simulink model "Uncoupled_Aircraft_State_Space"  (R2024b)
settings: Solver=VariableStepAuto  StartTime=0.0  StopTime=600  RelTol=1e-3
values from neighbouring files (symbols this model uses):
  A_lat = [ ... (first row only)    [Rigid_Aircraft_Simulink_Initializer.m]    (also in initialize_plane.m)
  A_long = [ ... (first row only)    [Rigid_Aircraft_Simulink_Initializer.m]    (also in initialize_plane.m)
  B_lat = [ B_ail , B_rud]    [Rigid_Aircraft_Simulink_Initializer.m]    (also in initialize_plane.m)
  B_long = [  B_elv , B_thr ]    [Rigid_Aircraft_Simulink_Initializer.m]    (also in initialize_plane.m)
  const_wind_vector = [6;0;0]    [Rigid_Aircraft_Simulink_Initializer.m]    (also in initialize_plane.m)
  energy_factor_lookup = readmatrix('Energy_Factor_Lookup.csv')    [Rigid_Aircraft_Simulink_Initializer.m]    (also in initialize_plane.m)
  init_alt = 20    [Rigid_Aircraft_Simulink_Initializer.m]    (also in initialize_plane.m = 60)
  init_lat = 52    [Rigid_Aircraft_Simulink_Initializer.m]    (also in initialize_plane.m = 51)
  init_long = 0    [Rigid_Aircraft_Simulink_Initializer.m]    (also in initialize_plane.m)
  L1 = 100    [Rigid_Aircraft_Simulink_Initializer.m]    (also in initialize_plane.m)
  L_day = 25    [Rigid_Aircraft_Simulink_Initializer.m]    (also in initialize_plane.m = 27)
  L_hr = 8    [Rigid_Aircraft_Simulink_Initializer.m]    (also in initialize_plane.m)
  L_month = 8    [Rigid_Aircraft_Simulink_Initializer.m]    (also in initialize_plane.m)
  L_year = 2025    [Rigid_Aircraft_Simulink_Initializer.m]    (also in initialize_plane.m)
  lap_tog = 0    [Rigid_Aircraft_Simulink_Initializer.m]    (also in initialize_plane.m)
  laps = 1    [Rigid_Aircraft_Simulink_Initializer.m]    (also in initialize_plane.m = 10)
  max_cap = 3600*236.80    (= 852480)    [Rigid_Aircraft_Simulink_Initializer.m]    (also in initialize_plane.m)
  max_power_income = 1100*0.18*0.46208    (= 91.49184)    [Rigid_Aircraft_Simulink_Initializer.m]    (also in initialize_plane.m)
  MG = readmatrix('METEO_data.csv')    [Rigid_Aircraft_Simulink_Initializer.m]    (also in initialize_plane.m)
  MGs1 = nan(nlat, nlon, ntime)    [Rigid_Aircraft_Simulink_Initializer.m]    (also in initialize_plane.m)
  MGs2 = nan(nlat, nlon, ntime)    [Rigid_Aircraft_Simulink_Initializer.m]    (also in initialize_plane.m)
  MGs3 = nan(nlat, nlon, ntime)    [Rigid_Aircraft_Simulink_Initializer.m]    (also in initialize_plane.m)
  MGs4 = nan(nlat, nlon, ntime)    [Rigid_Aircraft_Simulink_Initializer.m]    (also in initialize_plane.m)
  MGs5 = nan(nlat, nlon, ntime)    [Rigid_Aircraft_Simulink_Initializer.m]    (also in initialize_plane.m)
  MGs6 = nan(nlat, nlon, ntime)    [Rigid_Aircraft_Simulink_Initializer.m]    (also in initialize_plane.m)
  motor_power = 300    [Rigid_Aircraft_Simulink_Initializer.m]    (also in initialize_plane.m)
  u_trim = xu_trim(5:6)    [Rigid_Aircraft_Simulink_Initializer.m]    (also in initialize_plane.m)
  wind_tog = 1    [Rigid_Aircraft_Simulink_Initializer.m]    (also in initialize_plane.m)
  wind_type = 1    [Rigid_Aircraft_Simulink_Initializer.m]    (also in initialize_plane.m)
  wp_rad = 50    [Rigid_Aircraft_Simulink_Initializer.m]    (also in initialize_plane.m)
  wpts = wpts + zeros(6,1)    [A_star_IP.m]    (also in Rigid_Aircraft_Simulink_Initializer.m = wpts(:,2:end))
  X_eq = [U_inf; 0; 0; Theta_eq]    [Rigid_Aircraft_Simulink_Initializer.m]    (also in initialize_plane.m)
undefined symbols (not defined in the file or in its folder): Alt, aspd_min, gravity, H_INIT, K_D, K_H, K_T, K_V, mass, PTCH2SRV_D, PTCH2SRV_RLL, PTCH2SRV_RMAX_DN, PTCH2SRV_RMAX_UP, PTCH2SRV_TCONST, PTCH_K_I, PTCH_K_P, RLL2SRV_D, RLL2SRV_MAX, RLL2SRV_TCONST, RLL_K_I, RLL_K_P, V_INIT, YAW2SRV_DAMP, YAW2SRV_INT, YAW2SRV_RLL, YAW2SRV_SLIP
libraries: simulink_extras x19, eeGeneralControl x3, dspsrcs4 x3, dspswit3 x2, slpidlib x1, dspstat3 x1, simulink x1
settings Model: Creator=sh2323  LastModifiedBy=sh2323

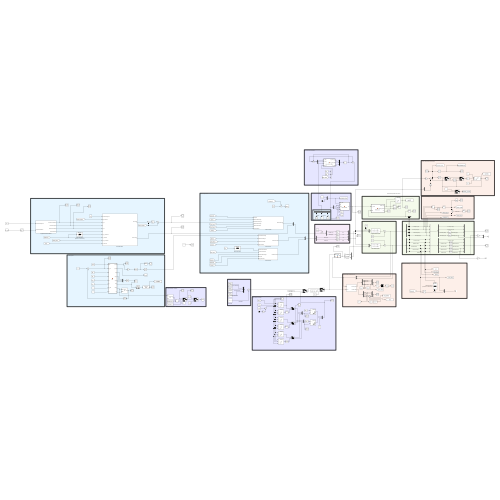
[thumbnail: Simulink's stored preview of the top-level diagram]
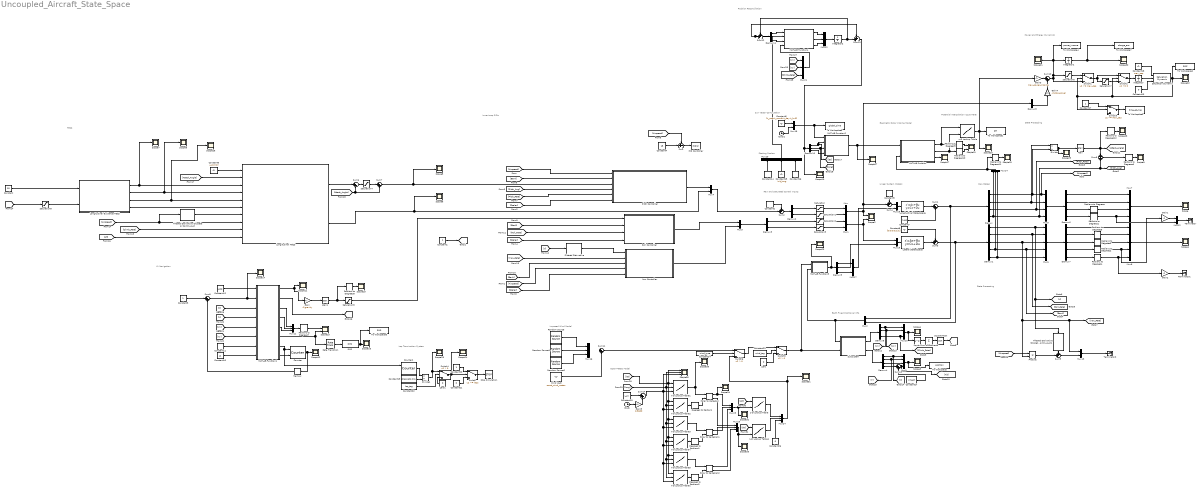
== system Uncoupled_Aircraft_State_Space ==
  note: Potential Interpolation Issue Here!
  note: Open-Meteo Model
  note: Imposed Wind Model
  note: Position Reconciliation
  note: Starting Positon
  note: Power and Energy Dynamics
  note: Lap Termination System
  note: Sun Vector Computation
  note: Geometric Solar Income Model
  note: L1 Navigation
  note: State Processing
  note: State Processing
  note: TECS
  note: Earth Fixed Positional Info
  note: Inner Loop PIDs
  note: Linear System Models
  note: Raw States
  note: Raw and Saturated Control Inputs
  1-D Lookup Table : Lookup_n-D  NumberOfTableDimensions=1  BreakpointsForDimension1=[10;80;120]  TableSource=Input port  Table=Alt  InterpMethod=Cubic spline  ExtrapMethod=Clip  InternalRulePriority=Speed  RndMeth=Simplest
      settings: InputPortMap=u0,p221
  1-D Lookup Table1 : Lookup_n-D  NumberOfTableDimensions=1  BreakpointsForDimension1=[10;80;120]  TableSource=Input port  Table=Alt  InterpMethod=Cubic spline  ExtrapMethod=Clip  InternalRulePriority=Speed  RndMeth=Simplest
      settings: InputPortMap=u0,p221
  Atan : Trigonometry  Operator=atan
  Atan1 : Trigonometry  Operator=atan
  Clock : Clock
  Clock1 : Clock
  Constant : Constant  Value=15
  Constant{1,3,17,20} (4 alike) : Constant
  Constant10 : Constant  Value=L1
  Constant11 : Constant  Value=wp_rad
  Constant12 : Constant  Value=wpts  VectorParams1D=off
  Constant13 : Constant  Value=0
  Constant14 : Constant  Value=init_lat
  Constant15 : Constant  Value=init_long
  Constant16 : Constant  Value=init_alt
  Constant18 : Constant  Value=max_cap
  Constant19 : Constant  Value=size(wpts,2)-1
  Constant2 : Constant  Value=u_trim
  Constant21 : Constant  Value=0
  Constant22 : Constant  Value=lap_tog
  Constant23 : Constant  Value=wind_tog
  Constant24 : Constant  Value=wind_type
  Constant25 : Constant  Value=L_hr
  Constant26 : Constant  Value=0
  Constant27 : Constant  Value=init_alt
  Constant4 : Constant  Value=15
  Constant5 : Constant  Value=[L_year;L_month;L_day;L_hr;0]
  Constant6 : Constant  Value=u_trim(2)
  Constant7 : Constant  Value=X_eq
  Constant8 : Constant  Value=[0;0;0;0;pi/2]
  Constant9 : Constant  Value=u_trim
  Counter : dspswit3/Counter  Direction=Up  CountEvent=Rising edge  CounterSize=User defined  MaxCount=255  InitialCount=0  Output=Count  HitValue=32  ResetInput=on  SamplesPerFrame=1  Ts=1  CntDtype=double  HitDtype=Logical
  Counter1 : dspswit3/Counter  Direction=Up  CountEvent=Rising edge  CounterSize=User defined  MaxCount=255  InitialCount=0  Output=Count  HitValue=32  ResetInput=on  SamplesPerFrame=1  Ts=1  CntDtype=double  HitDtype=Logical
  Degrees to Radians : simulink_extras/Transformations/Degrees to Radians
  Degrees to Radians1 : simulink_extras/Transformations/Degrees to Radians
  Degrees to Radians2 : simulink_extras/Transformations/Degrees to Radians
  Demux{,4..6} (4 alike) : Demux
  Demux1 : Demux  Outputs=5
  Demux10 : Demux  Outputs=3
  Demux11 : Demux  Outputs=3
  Demux2 : Demux  Outputs=2
  Demux3 : Demux  Outputs=2
  Demux7 : Demux  Outputs=5
  Demux8 : Demux  Outputs=2
  Demux9 : Demux  Outputs=3
  Divide : Product  Inputs=*/
  Divide1 : Product  Inputs=*/
  "Filtered Derivative " : eeGeneralControl/Filtered Derivative (Discrete or Continuous)  K=1  T=0.1  B=inf  A=-inf  minRatio=10  init_option=Inherited from block input  x0=0  Ts=-1
      settings: LibrarySourceBlock=|
      | ee_sl_lib/General Control/Filtered Derivative
      | (Discrete or Continuous)
  Filtered Derivative (Discrete or Continuous) : eeGeneralControl/Filtered Derivative (Discrete or Continuous)  K=1  T=0.1  B=inf  A=-inf  minRatio=10  init_option=Inherited from block input  x0=0  Ts=-1
      settings: LibrarySourceBlock=|
      | ee_sl_lib/General Control/Filtered Derivative
      | (Discrete or Continuous)
  Filtered Derivative (Discrete or Continuous)1 : eeGeneralControl/Filtered Derivative (Discrete or Continuous)  K=1  T=0.1  B=inf  A=-inf  minRatio=10  init_option=Inherited from block input  x0=0  Ts=-1
      settings: LibrarySourceBlock=|
      | ee_sl_lib/General Control/Filtered Derivative
      | (Discrete or Continuous)
  Gain : Gain  Gain=-1/gravity
  Gain1 : Gain  Gain=-1
  Gain2 : Gain  Gain=-1
  Gain3 : Gain  Gain=max_power_income
  Gain4 : Gain  Gain=-motor_power
  Gain5 : Gain  Gain=1/3600
  Integrator : Integrator  InitialCondition=max_cap
  Integrator1 : Integrator
  Integrator2 : Integrator
  Lateral State-Space : StateSpace  A=A_lat  B=[B_lat A_lat(:,1)]  C=eye(5)  D=zeros(size([B_lat A_lat(:,1)]))  InitialCondition=0
  Longitudinal Guidance TECS : Subsystem
  Longitudinal State-Space : StateSpace  A=A_long  B=[B_long A_long(:,1:2)]  C=eye(4)  D=zeros(size([B_long A_long(:,1:2)]))  InitialCondition=0
  Longitudinal TECS : Subsystem
  MATLAB Function : MATLAB Function  TreatAsAtomicUnit=on
  MATLAB Function1 : MATLAB Function  TreatAsAtomicUnit=on
  MATLAB Function2 : MATLAB Function  TreatAsAtomicUnit=on
  MATLAB Function3 : MATLAB Function  TreatAsAtomicUnit=on
  MATLAB Function4 : MATLAB Function  TreatAsAtomicUnit=on
  Memory : Memory
  Mux{,1..4,12..13,15,17..19} (11 alike) : Mux  Inputs=2
  Mux{5,7,9..10} (4 alike) : Mux
  Mux{11,14,16,20..25} (9 alike) : Mux  Inputs=3
  Mux6 : Mux  Inputs=5
  Mux8 : Mux  Inputs=5
  PID Controller : slpidlib/PID Controller  Controller=PID  Form=Parallel  TimeDomain=Continuous-time  UseExternalTs=off  SampleTime=-1  IntegratorMethod=Forward Euler  FilterMethod=Forward Euler  ControllerParametersSource=internal  P=1  I=1  UseKiTs=off  D=0  UseExternalDerivativeSource=off  N=100  UseFilter=on  TunerSelectOption=Transfer Function Based (PID Tuner App)  InitialConditionSource=internal  InitialConditionForIntegrator=0  InitialConditionForFilter=0  DifferentiatorICPrevScaledInput=0  ExternalReset=none  TrackingMode=off  Kt=1  LimitOutput=off  SatLimitsSource=internal  UpperSaturationLimit=inf  LowerSaturationLimit=-inf  LinearizeAsGain=on  AntiWindupMode=none  Kb=1  LimitIntegrator=off  UpperIntegratorSaturationLimit=inf  LowerIntegratorSaturationLimit=-inf  POutMin=[]  POutMax=[]  IOutMin=[]  IOutMax=[]  DOutMin=[]  DOutMax=[]  NOutMin=[]  NOutMax=[]  SumOutMin=[]  SumOutMax=[]  SaturationOutMin=[]  SaturationOutMax=[]  PParamMin=[]  PParamMax=[]  IParamMin=[]  IParamMax=[]  DParamMin=[]  DParamMax=[]  NParamMin=[]  NParamMax=[]  KbParamMin=[]  KbParamMax=[]  KtParamMin=[]  KtParamMax=[]  KbOutMin=[]  KbOutMax=[]  KtOutMin=[]  KtOutMax=[]  IntegratorOutMin=[]  IntegratorOutMax=[]  FilterOutMin=[]  FilterOutMax=[]  SumI1OutMin=[]  SumI1OutMax=[]  SumI2OutMin=[]  SumI2OutMax=[]  SumI3OutMin=[]  SumI3OutMax=[]  SumI4OutMin=[]  SumI4OutMax=[]  SumDOutMin=[]  SumDOutMax=[]  DifferentiatorOutMin=[]  DifferentiatorOutMax=[]  FilterDiffOutCoefMin=[]  FilterDiffOutCoefMax=[]  ReciprocalOutMin=[]  ReciprocalOutMax=[]  SumDenOutMin=[]  SumDenOutMax=[]  SumNumOutMin=[]  SumNumOutMax=[]  DivideOutMin=[]  DivideOutMax=[]  UdiffTsProdOutMin=[]  UdiffTsProdOutMax=[]  NTsProdOutMin=[]  NTsProdOutMax=[]  UintegralTsProdOutMin=[]  UintegralTsProdOutMax=[]  UngainTsProdOutMin=[]  UngainTsProdOutMax=[]  ClampingZeroOutDataTypeStr=Inherit: Inherit via back propagation  ClampingZeroOutMin=[]  ClampingZeroOutMax=[]  FilterDenConstantOutDataTypeStr=Inherit: Inherit via back propagation  FilterDenConstantOutMin=[]  FilterDenConstantOutMax=[]  PCopyOutDataTypeStr=Inherit: Inherit via back propagation  PCopyOutMin=[]  PCopyOutMax=[]  NCopyOutDataTypeStr=Inherit: Inherit via back propagation  NCopyOutMin=[]  NCopyOutMax=[]  IntegratorContinuousStateAttributes=''  IntegratorStateMustResolveToSignalObject=off  IntegratorRTWStateStorageClass=Auto  FilterContinuousStateAttributes=''  FilterStateMustResolveToSignalObject=off  FilterRTWStateStorageClass=Auto  ParallelPVariant=InternalParameters  IdealPVariant=Disabled  IVariant=InternalParameters  DVariant=InternalParameters  IntegratorVariant=Continuous  SatVariant=Disabled  AWVariant=Passthrough  PCopyVariant=Disabled  TRVariant=Disabled  FdbkBlocksVariant=Forward  IdealPFdbkVariant=Disabled  SatFdbkVariant=Disabled  DerivativeFilterVariant=ContFilter  NVariant=InternalParameters  NCopyVariant=Disabled  FilterICVariant=InternalICsFilter  IntegratorICVariant=InternalICs  ExternalResetVariant=Disabled  TRSumVariant=Passthrough  SumFdbkVariant=Disabled  SumVariant=Sum_PID  TsampFilterVariant=InternalTs  TsampNgainVariant=Passthrough  TsampIntegralVariant=Disabled_SignalSpec  ExternalSaturationOutDataTypeStr=Inherit: Same as second input  DerivativeSourceVariant=ErrorSignal  PreIntVariant=InternalPreInt
  Pitch Controller : Subsystem
  Polar to Cartesian : simulink_extras/Transformations/Polar to Cartesian
  Polar to Cartesian1 : simulink_extras/Transformations/Polar to Cartesian
  Polar to Cartesian2 : simulink_extras/Transformations/Polar to Cartesian
  Product : Product
  RMS : dspstat3/RMS  run=on  directionMode=Each column  dimension=1  InputProcessing=Columns as channels (frame based)  reset_popup=None
  Radians to Degrees{,1..12} (13 alike) : simulink_extras/Transformations/Radians to Degrees
  Random Source : dspsrcs4/Random Source  SrcType=Gaussian  MinVal=0  MaxVal=1  MeanVal=0  VarVal=0  RepMode=Specify seed  rawSeed=1  IsInherit=off  SampTime=0.25  SampFrame=1  OutComplex=Real  DataType=double  SimulateUsing=Interpreted execution
  Random Source1 : dspsrcs4/Random Source  SrcType=Gaussian  MinVal=0  MaxVal=1  MeanVal=0  VarVal=0.1  RepMode=Specify seed  rawSeed=1  IsInherit=off  SampTime=0.25  SampFrame=1  OutComplex=Real  DataType=double  SimulateUsing=Interpreted execution
  Random Source2 : dspsrcs4/Random Source  SrcType=Gaussian  MinVal=0  MaxVal=1  MeanVal=0  VarVal=0.01  RepMode=Specify seed  rawSeed=1  IsInherit=off  SampTime=0.25  SampFrame=1  OutComplex=Real  DataType=double  SimulateUsing=Interpreted execution
  Rate Transition : RateTransition  OutPortSampleTime=0.05
  Roll Controller : Subsystem
  Saturation : Saturate  UpperLimit=1  LowerLimit=-1
  Saturation Dynamic : simulink/Discontinuities/Saturation Dynamic  OutMin=[]  OutMax=[]  OutDataTypeStr=Inherit: Same as second input  OutDataType=fixdt(1, 16)  OutScaling=2^-10  DoSatur=off
  Saturation1 : Saturate  UpperLimit=1  LowerLimit=0
  Saturation2 : Saturate  UpperLimit=1  LowerLimit=-1
  Saturation3 : Saturate  UpperLimit=1  LowerLimit=-1
  Saturation4 : Saturate  UpperLimit=deg2rad(10)  LowerLimit=deg2rad(-10)
  Saturation5 : Saturate  UpperLimit=deg2rad(30)  LowerLimit=-deg2rad(30)
  Saturation6 : Saturate  UpperLimit=0  LowerLimit=-inf
  Saturation7 : Saturate  UpperLimit=inf  LowerLimit=0
  Saturation8 : Saturate  UpperLimit=120  LowerLimit=0
  Scope{,1,3..9,11..12,14..35} (33 alike) : Scope
  Scope10 : Scope  NumInputPorts=2
  Scope13 : Scope  NumInputPorts=2
  Scope2 : Scope  NumInputPorts=2
  Scope36 : Scope  NumInputPorts=3
  Square : Math  Operator=square
  Square Root : Sqrt
  Stop Simulation : Stop
  Subsystem : Subsystem
  Sum : Sum  Inputs=-+|
  Sum of Elements : Sum  Inputs=+
  Sum{1,7..8,10..11,14..15} (7 alike) : Sum  Inputs=|++
  Sum{2..3,9,12..13} (5 alike) : Sum  Inputs=++|
  Sum4 : Sum  Inputs=-+|
  Sum5 : Sum  Inputs=+|+
  Sum6 : Sum  Inputs=|+-
  Switch : Switch  Threshold=laps  SaturateOnIntegerOverflow=off  InputSameDT=off
  Switch1 : Switch  Threshold=max_cap  SaturateOnIntegerOverflow=off  InputSameDT=off
  Switch2 : Switch  SaturateOnIntegerOverflow=off  InputSameDT=off
  Switch3 : Switch  Threshold=max_cap  SaturateOnIntegerOverflow=off  InputSameDT=off
  Switch4 : Switch  Criteria=u2 > Threshold  SaturateOnIntegerOverflow=off  InputSameDT=off
  Switch5 : Switch  Criteria=u2 > Threshold  SaturateOnIntegerOverflow=off  InputSameDT=off
  Switch6 : Switch  Criteria=u2 > Threshold  SaturateOnIntegerOverflow=off  InputSameDT=off
  Terminator : Terminator
  Terminator1 : Terminator
  Terminator2 : Terminator
  To Workspace : ToWorkspace  VariableName=position  SaveFormat=Timeseries  SampleTime=-1
  To Workspace1 : ToWorkspace  VariableName=SFI  SaveFormat=Timeseries  SampleTime=-1
  To Workspace2 : ToWorkspace  VariableName=SOC  SaveFormat=Timeseries  SampleTime=-1
  To Workspace3 : ToWorkspace  VariableName=time_at_max  SaveFormat=Timeseries  SampleTime=-1
  To Workspace4 : ToWorkspace  VariableName=power_income  SaveFormat=Timeseries  SampleTime=-1
  To Workspace5 : ToWorkspace  VariableName=global_time  SaveFormat=Timeseries  SampleTime=-1
  To Workspace6 : ToWorkspace  VariableName=RMS  SaveFormat=Timeseries  SampleTime=-1
  To Workspace7 : ToWorkspace  VariableName=charge_acc  SaveFormat=Timeseries  SampleTime=-1
  Wind Vect : Constant  Value=const_wind_vector
  Yaw Controller : Subsystem
  Zero : Constant  Value=0  OutDataTypeStr=Inherit: Inherit via back propagation
  Zero1 : Constant  Value=0  OutDataTypeStr=Inherit: Inherit via back propagation
  n-D Lookup Table : Lookup_n-D  BreakpointsForDimension1=unique(energy_factor_lookup(:,1))  BreakpointsForDimension2=unique(energy_factor_lookup(:,2))  BreakpointsForDimension3=[5, 7]  Table=Z'  ExtrapMethod=Clip  InternalRulePriority=Speed  RndMeth=Simplest
      settings: InputPortMap=u0,u1
  n-D Lookup Table1 : Lookup_n-D  NumberOfTableDimensions=3  BreakpointsForDimension1=unique(MG(:,1))  BreakpointsForDimension2=unique(MG(:,2))  BreakpointsForDimension3=unique(MG(:,3))  Table=MGs1  InterpMethod=Cubic spline  ExtrapMethod=Clip  InternalRulePriority=Speed  RndMeth=Simplest
      settings: InputPortMap=u0,u1,u2
  n-D Lookup Table2 : Lookup_n-D  NumberOfTableDimensions=3  BreakpointsForDimension1=unique(MG(:,1))  BreakpointsForDimension2=unique(MG(:,2))  BreakpointsForDimension3=unique(MG(:,3))  Table=MGs2  InterpMethod=Cubic spline  ExtrapMethod=Clip  InternalRulePriority=Speed  RndMeth=Simplest
      settings: InputPortMap=u0,u1,u2
  n-D Lookup Table3 : Lookup_n-D  NumberOfTableDimensions=3  BreakpointsForDimension1=unique(MG(:,1))  BreakpointsForDimension2=unique(MG(:,2))  BreakpointsForDimension3=unique(MG(:,3))  Table=MGs3  InterpMethod=Cubic spline  ExtrapMethod=Clip  InternalRulePriority=Speed  RndMeth=Simplest
      settings: InputPortMap=u0,u1,u2
  n-D Lookup Table4 : Lookup_n-D  NumberOfTableDimensions=3  BreakpointsForDimension1=unique(MG(:,1))  BreakpointsForDimension2=unique(MG(:,2))  BreakpointsForDimension3=unique(MG(:,3))  Table=MGs4  InterpMethod=Cubic spline  ExtrapMethod=Clip  InternalRulePriority=Speed  RndMeth=Simplest
      settings: InputPortMap=u0,u1,u2
  n-D Lookup Table5 : Lookup_n-D  NumberOfTableDimensions=3  BreakpointsForDimension1=unique(MG(:,1))  BreakpointsForDimension2=unique(MG(:,2))  BreakpointsForDimension3=unique(MG(:,3))  Table=MGs5  InterpMethod=Cubic spline  ExtrapMethod=Clip  InternalRulePriority=Speed  RndMeth=Simplest
      settings: InputPortMap=u0,u1,u2
  n-D Lookup Table6 : Lookup_n-D  NumberOfTableDimensions=3  BreakpointsForDimension1=unique(MG(:,1))  BreakpointsForDimension2=unique(MG(:,2))  BreakpointsForDimension3=unique(MG(:,3))  Table=MGs6  InterpMethod=Cubic spline  ExtrapMethod=Clip  InternalRulePriority=Speed  RndMeth=Simplest
      settings: InputPortMap=u0,u1,u2
  wires:
  Demux7/5 -> Radians to Degrees4/1  "Heading (rad)"
  Demux1/5 -> Mux6/5, Mux14/3  "Heading (rad)"
  Mux6/1 -> Demux7/1
  Demux6/1 -> Mux7/1  "X-velocity U (m/s)"
  Demux/3 -> Mux5/3, [Pitch_Rate]  "Pitch Rate (rad/s)"
  Demux7/2 -> Radians to Degrees5/1  "Roll Rate (rad/s)"
  Radians to Degrees2/1 -> Gain1/1, Mux8/4  "Bank Angle (deg)"
  Mux5/1 -> Demux6/1
  Demux/4 -> Sum5/2, [Pitch_Ang], Mux5/4, Mux14/1  "Pitch Angle (rad)"
  Demux6/4 -> Radians to Degrees1/1  "Pitch Angle (rad)"
  Demux7/3 -> Radians to Degrees3/1  "Yaw Rate (rad/s)"
  Demux/2 -> Divide/1, Mux5/2  "Z-velocity  W (m/s)"
  Demux7/1 -> Mux8/1  "Y-velocity V (m/s)"
  Radians to Degrees/1 -> Mux7/3  "Pitch Rate (deg/s)"
  Demux1/2 -> [Roll_Rate], Mux6/2  "Roll Rate (rad/s)"
  Demux/1 -> Divide/2, [Airspeed], Mux5/1  "X-velocity U (m/s)"
  Radians to Degrees4/1 -> Gain2/1, Mux8/5  "Heading (deg)"
  Demux7/4 -> Radians to Degrees2/1  "Bank Angle (rad)"
  Demux1/1 -> [V], Filtered Derivative (Discrete or Continuous)1/1, Mux6/1  "Y-velocity V (m/s)"
  Radians to Degrees5/1 -> Mux8/2  "Roll Rate (deg/s)"
  Demux1/3 -> Product/2, Mux13/1, [Yaw_Rate], Mux6/3  "Yaw Rate (rad/s)"
  Demux6/3 -> Radians to Degrees/1  "Pitch Rate (rad/s)"
  Demux6/2 -> Mux7/2  "Z-velocity  W (m/s)"
  Mux8/1 -> Scope1/1
  Mux7/1 -> Scope/1
  Demux1/4 -> [Bank], Mux6/4, Mux14/2  "Bank Angle (rad)"
  Radians to Degrees3/1 -> Mux8/3  "Yaw Rate (deg/s)"
  Radians to Degrees1/1 -> Mux12/2, Mux7/4  "Pitch Angle (deg)"
  Lateral State-Space/1 -> Sum3/2
  Demux3/2 -> Saturation3/1  "Rudder(%)"
  Saturation1/1 -> Mux/2  "Thr"
  Saturation/1 -> Mux/1  "Elv"
  Demux2/1 -> Saturation/1  "Elelvator (%)"
  Demux3/1 -> Saturation2/1  "Aileron (%)"
  Saturation2/1 -> Mux1/1  "Ail"
  Demux2/2 -> Saturation1/1  "Throttle (%)"
  Saturation3/1 -> Mux1/2  "Rud"
  Mux/1 -> Sum4/2, Demux8/1, Scope2/1
  Mux1/1 -> Mux19/1, Scope2/2
  Sum2/1 -> Demux2/1
  Longitudinal State-Space/1 -> Sum1/1
  Mux2/1 -> MATLAB Function3/2(X), Subsystem/1(X)
  Mux4/1 -> Sum2/2
  Mux3/1 -> Demux3/1
  Roll Controller/1(Aileron Demand) -> Mux3/1
  Yaw Controller/1(Rudder Demand) -> Mux3/2
  "Filtered Derivative "/1 -> Yaw Controller/1(Measured Acceleration)
  Sum/1 -> PID Controller/1
  Constant4/1 -> Sum/2
  Pitch Controller/1(Elevator Demand) -> Mux4/1
  Longitudinal Guidance TECS/4(Desired Altitude) -> Longitudinal TECS/6(h)
  Longitudinal Guidance TECS/3(Desired Climb Rate) -> Scope26/1, Longitudinal TECS/5(h_dot)
  [Climb_Rate] -> Longitudinal TECS/9(h_dot_measured)
  Longitudinal Guidance TECS/2(Desired Airspeed) -> Scope8/1, Longitudinal TECS/4(V)
  Longitudinal Guidance TECS/1(Desired Acceleration) -> Scope7/1, Longitudinal TECS/3(V_dot)
  Constant/1 -> Longitudinal Guidance TECS/1(Commanded Airspeed)
  [Alt] -> Longitudinal TECS/10(h_measured)
  [Airspeed] -> Pitch Controller/1(Airspeed)
  [Airspeed] -> Yaw Controller/4(Airspeed)
  Constant1/1 -> [Scaler]
  [Scaler] -> Pitch Controller/6(Airspeed Scaler)
  [Scaler] -> Roll Controller/4(Airspeed Scaler)
  [Scaler] -> Yaw Controller/5(Airspeed Scaler)
  [Airspeed] -> Sum/1
  [Pitch_Ang] -> Pitch Controller/4(Measured Pitch Angle)
  [Pitch_Rate] -> Pitch Controller/5(Measured Pitch Rate)
  [Bank] -> Pitch Controller/2(Measured Bank Angle)
  [Bank] -> Roll Controller/2(Measured Roll Angle)
  [Bank] -> Yaw Controller/3(Measured Bank Angle)
  [Roll_Rate] -> Roll Controller/3(Measured Roll Rate)
  [V] -> "Filtered Derivative "/1
  [Yaw_Rate] -> Yaw Controller/2(Measured Yaw Rate)
  Sum1/1 -> Mux2/1, Demux/1
  Sum3/1 -> Demux1/1, Mux2/2
  Constant7/1 -> Sum1/2
  Constant8/1 -> Sum3/1
  Constant2/1 -> Sum2/1
  Subsystem/2(Position Vec) -> Demux4/1
  Subsystem/1(Velocity Vec.) -> Demux5/1
  Demux5/1 -> Mux10/1, [Vx]  "X-Velocity (m/s)"
  Demux5/2 -> Mux10/2, [Vy]  "Y-Velocity (m/s)"
  Demux5/4 -> [Climb_Rate], Mux10/4  "Climb Rate (m/s)"
  Mux10/1 -> Square/1, Scope4/1
  Demux4/2 -> [Y], Mux9/2  "Y (m)"
  Mux9/1 -> To Workspace/1, Scope3/1
  Square/1 -> Sum of Elements/1
  Sum of Elements/1 -> Square Root/1
  Square Root/1 -> [V_net]
  [Airspeed] -> Longitudinal TECS/8(V_measured), Filtered Derivative (Discrete or Continuous)/1
  Filtered Derivative (Discrete or Continuous)/1 -> Longitudinal TECS/7(V_dot_measured)
  Divide/1 -> Scope29/1, Atan/1
  Atan/1 -> Radians to Degrees12/1, Sum5/1, [Attack_Angle]
  Longitudinal TECS/2(Thrust Control) -> Scope6/1, Mux4/2
  Longitudinal TECS/1(Pitch Angle) -> Sum6/1
  Sum5/1 -> Radians to Degrees6/1  "Climb Grad."
  Radians to Degrees6/1 -> Scope9/1
  Constant6/1 -> Longitudinal TECS/1(estimated drag force)
  Sum7/1 -> Scope5/1, Pitch Controller/3(Demanded Pitch Angle)
  Sum6/1 -> Saturation4/1
  Saturation4/1 -> Sum7/1
  MATLAB Function1/1(a_cmd) -> Gain/1, Scope11/1
  Constant11/1 -> MATLAB Function1/7(wp_rad)
  Demux4/1 -> [X], Mux9/1  "X (m)"
  [Y] -> MATLAB Function1/4(Y)
  [Vx] -> MATLAB Function1/5(Vx)
  [Vy] -> MATLAB Function1/6(Vy)
  Constant12/1 -> MATLAB Function1/1(wpts)
  Gain/1 -> Atan1/1
  MATLAB Function1/3(ang) -> Mux11/1
  Radians to Degrees7/1 -> Scope13/1
  Radians to Degrees8/1 -> Scope15/1
  Atan1/1 -> Saturation5/1, Radians to Degrees8/1
  Demux4/3 -> Mux9/3
  [X] -> MATLAB Function1/3(X)
  Constant10/1 -> MATLAB Function1/8(L1)
  Counter/1 -> Memory/1, Scope12/1
  MATLAB Function1/7(ticker) -> Counter1/1, Counter/1
  Sum8/1 -> Scope14/1, MATLAB Function1/2(wp_id)
  Constant3/1 -> Sum8/1
  Memory/1 -> Sum8/2
  MATLAB Function1/4(eta_1) -> Mux11/2
  MATLAB Function1/5(eta_2) -> Mux11/3
  Mux11/1 -> Radians to Degrees7/1
  MATLAB Function1/6(CTE) -> Rate Transition/1, Scope13/2
  RMS/1 -> To Workspace6/1, Scope16/1
  Rate Transition/1 -> RMS/1
  Mux12/1 -> Terminator/1
  Gain1/1 -> Mux12/1
  Gain2/1 -> Terminator1/1
  [Airspeed] -> Product/1
  Product/1 -> Sum9/2
  Filtered Derivative (Discrete or Continuous)1/1 -> Sum9/1
  Sum9/1 -> Mux13/2
  Mux13/1 -> Terminator2/1
  MATLAB Function1/2(h_cmd) -> [h_cmd]
  MATLAB Function1/8(rst) -> Counter/2
  MATLAB Function2/1(SI) -> Scope27/1, MATLAB Function/1(sun_vector)
  MATLAB Function/1(relative_elv) -> n-D Lookup Table/1, Radians to Degrees9/1
  MATLAB Function/2(relative_azimuth) -> n-D Lookup Table/2, Radians to Degrees10/1
  Radians to Degrees9/1 -> Scope10/1
  Radians to Degrees10/1 -> Scope10/2
  MATLAB Function/3(vec) -> Scope17/1
  Constant5/1 -> Mux15/1
  Clock1/1 -> Mux15/2
  n-D Lookup Table/1 -> Gain3/1, Scope20/1, To Workspace1/1
  Demux8/2 -> Gain4/1
  Gain4/1 -> Sum10/2
  Gain3/1 -> Sum10/1
  Integrator/1 -> Saturation Dynamic/2
  Saturation Dynamic/1 -> To Workspace2/1, Switch1/2, Switch3/2, Switch2/2, Scope22/1
  Constant13/1 -> Saturation Dynamic/3
  Saturation6/1 -> Switch1/1
  Sum10/1 -> Switch1/3, Scope21/1, To Workspace4/1, Integrator1/1, Saturation6/1
  Switch2/1 -> Integrator/1
  Switch1/1 -> Switch2/1, Saturation7/1
  Saturation7/1 -> Switch2/3
  Constant18/1 -> Saturation Dynamic/1
  Constant17/1 -> Switch3/1
  Switch3/1 -> To Workspace3/1
  Random Source/1 -> Mux16/1  "North wind Noise"
  Random Source1/1 -> Mux16/2  "East Wind Noise"
  Random Source2/1 -> Mux16/3  "Down Wind Noise"
  Wind Vect/1 -> Sum11/2  "NED Wind"
  MATLAB Function3/1(Wind) -> Scope23/1, Demux9/1
  Constant9/1 -> Sum4/1
  Mux18/1 -> Longitudinal State-Space/1
  Sum4/1 -> Mux18/1
  Demux9/1 -> Mux17/1  "U-wind"
  Mux19/1 -> Lateral State-Space/1
  Mux15/1 -> MATLAB Function2/1(time_info), To Workspace5/1
  Constant19/1 -> Divide1/2
  Switch/1 -> Stop Simulation/1
  Constant20/1 -> Switch/1
  Constant21/1 -> Switch/3
  Counter1/1 -> Divide1/1
  Switch4/1 -> Switch/2, Scope24/1
  Constant22/1 -> Switch4/2
  Divide1/1 -> Scope25/1, Switch4/1
  Integrator1/1 -> To Workspace7/1, Scope30/1
  Mux14/1 -> Radians to Degrees11/1, MATLAB Function/2(Euler)
  Radians to Degrees11/1 -> Scope18/1
  Radians to Degrees12/1 -> Scope28/1
  Demux9/2 -> Mux19/2  "V-wind"
  Demux9/3 -> Mux17/2  "W-wind"
  [Attack_Angle] -> Sum7/2, Sum6/2
  [Attack_Angle] -> Longitudinal TECS/2(angle of attack)
  Mux17/1 -> Mux18/2
  Constant14/1 -> Mux20/1  "latitude"
  Constant15/1 -> Mux20/2  "longitude"
  Demux10/1 -> [lat], MATLAB Function2/2(lat)
  Demux10/2 -> [long], MATLAB Function2/3(long)
  Demux10/3 -> MATLAB Function2/4(alt)
  Constant16/1 -> Mux20/3  "alt"
  Saturation5/1 -> Roll Controller/1(Demanded Roll Angle)
  Sum13/1 -> Scope19/1, Demux10/1
  Demux11/3 -> MATLAB Function4/3(h)
  Mux22/1 -> Integrator2/1
  MATLAB Function4/2(lon_rate_deg) -> Mux22/2
  MATLAB Function4/1(lat_rate_deg) -> Mux22/1
  [Vx] -> Mux21/1
  MATLAB Function4/3(h_rate) -> Mux22/3
  [Climb_Rate] -> Mux21/3
  [Vy] -> Mux21/2
  Mux21/1 -> MATLAB Function4/4(neu_vel)
  Integrator2/1 -> Sum13/2, Sum12/1
  Demux11/2 -> MATLAB Function4/2(lon_deg)
  Sum12/1 -> Demux11/1
  Mux20/1 -> Sum13/1, Sum12/2
  Demux11/1 -> MATLAB Function4/1(lat_deg)
  Switch5/1 -> MATLAB Function3/1(Earth_Wind), Subsystem/2(wind)
  Constant23/1 -> Switch5/2
  Switch6/1 -> Switch5/1
  Sum11/1 -> Switch6/1
  Constant24/1 -> Switch6/2
  n-D Lookup Table1/1 -> Scope35/1, Polar to Cartesian/1
  Zero/1 -> Switch5/3
  Zero1/1 -> Switch4/3
  [lat] -> Scope36/1, n-D Lookup Table6/1, n-D Lookup Table5/1, n-D Lookup Table4/1, n-D Lookup Table3/1, n-D Lookup Table2/1, n-D Lookup Table1/1
  [long] -> Scope36/2, n-D Lookup Table6/2, n-D Lookup Table5/2, n-D Lookup Table4/2, n-D Lookup Table3/2, n-D Lookup Table2/2, n-D Lookup Table1/2
  Constant25/1 -> Sum14/1
  Gain5/1 -> Sum14/2
  Clock/1 -> Gain5/1
  Sum14/1 -> Scope36/3, n-D Lookup Table6/3, n-D Lookup Table5/3, n-D Lookup Table4/3, n-D Lookup Table3/3, n-D Lookup Table2/3, n-D Lookup Table1/3
  n-D Lookup Table3/1 -> Polar to Cartesian1/1
  n-D Lookup Table5/1 -> Polar to Cartesian2/1
  Polar to Cartesian/1 -> Scope34/1, Mux23/1
  Polar to Cartesian1/1 -> Mux23/2
  Polar to Cartesian2/1 -> Mux23/3
  1-D Lookup Table/1 -> Mux24/1
  1-D Lookup Table1/1 -> Mux24/2
  Constant26/1 -> Mux24/3
  Polar to Cartesian1/2 -> Mux25/2
  Polar to Cartesian/2 -> Mux25/1
  Polar to Cartesian2/2 -> Mux25/3
  Mux25/1 -> 1-D Lookup Table1/2, Scope33/1
  Mux24/1 -> Scope31/1, Switch6/3
  n-D Lookup Table2/1 -> Degrees to Radians/1
  Degrees to Radians/1 -> Polar to Cartesian/2
  n-D Lookup Table4/1 -> Degrees to Radians1/1
  Degrees to Radians1/1 -> Polar to Cartesian1/2
  n-D Lookup Table6/1 -> Degrees to Radians2/1
  Degrees to Radians2/1 -> Polar to Cartesian2/2
  Mux23/1 -> 1-D Lookup Table/2, Scope32/1
  [Alt] -> 1-D Lookup Table/1
  [Alt] -> 1-D Lookup Table1/1
  Constant27/1 -> Sum15/2
  [h_cmd] -> Saturation8/1
  Saturation8/1 -> Longitudinal Guidance TECS/2(Commanded Altitude)
  Sum15/1 -> [Alt], Mux9/4
  Demux4/4 -> Sum15/1  "Alt (m)"

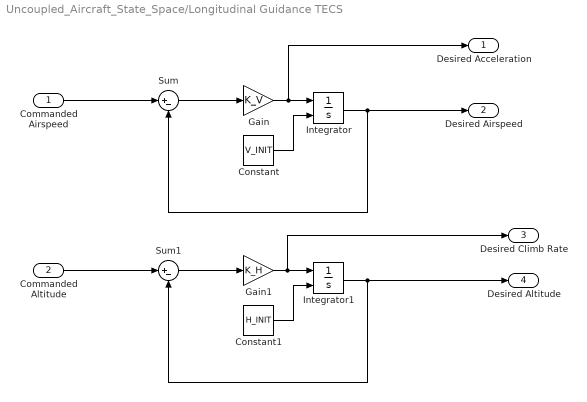
== system Uncoupled_Aircraft_State_Space/Longitudinal Guidance TECS ==
  Commanded Airspeed : Inport
  Commanded Altitude : Inport  Port=2
  Constant : Constant  Value=V_INIT
  Constant1 : Constant  Value=H_INIT
  Gain : Gain  Gain=K_V
  Gain1 : Gain  Gain=K_H
  Integrator : Integrator  InitialConditionSource=external
  Integrator1 : Integrator  InitialConditionSource=external
  Sum : Sum  Inputs=|+-
  Sum1 : Sum  Inputs=|+-
  Desired Acceleration : Outport
  Desired Airspeed : Outport  Port=2
  Desired Climb Rate : Outport  Port=3
  Desired Altitude : Outport  Port=4
  wires:
  Sum/1 -> Gain/1
  Gain/1 -> Desired Acceleration/1, Integrator/1
  Commanded Altitude/1 -> Sum1/1
  Constant/1 -> Integrator/2
  Integrator1/1 -> Desired Altitude/1, Sum1/2
  Gain1/1 -> Desired Climb Rate/1, Integrator1/1
  Commanded Airspeed/1 -> Sum/1
  Integrator/1 -> Desired Airspeed/1, Sum/2
  Constant1/1 -> Integrator1/2
  Sum1/1 -> Gain1/1

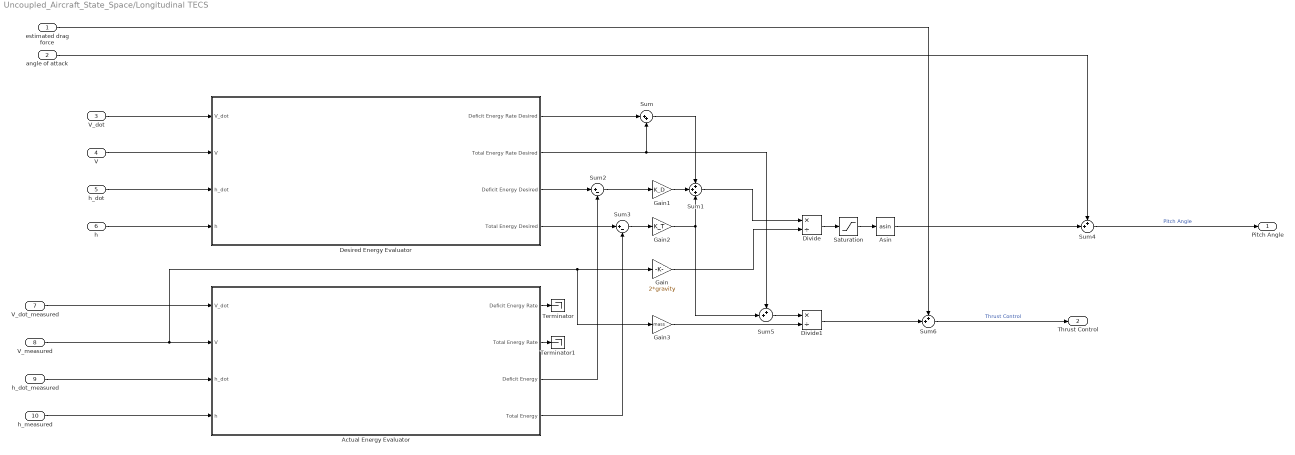
== system Uncoupled_Aircraft_State_Space/Longitudinal TECS ==
  estimated drag force : Inport
  angle of attack : Inport  Port=2
  V_dot : Inport  Port=3
  V : Inport  Port=4
  h_dot : Inport  Port=5
  h : Inport  Port=6
  V_dot_measured : Inport  Port=7
  V_measured : Inport  Port=8
  h_dot_measured : Inport  Port=9
  h_measured : Inport  Port=10
  Actual Energy Evaluator : Subsystem
  Asin : Trigonometry  Operator=asin
  Desired Energy Evaluator : Subsystem
  Divide : Product  Inputs=*/
  Divide1 : Product  Inputs=*/
  Gain : Gain  Gain=2*gravity
  Gain1 : Gain  Gain=K_D
  Gain2 : Gain  Gain=K_T
  Gain3 : Gain  Gain=mass
  Saturation : Saturate  UpperLimit=1  LowerLimit=-1
  Sum : Sum  Inputs=|++
  Sum1 : Sum  Inputs=+++
  Sum2 : Sum  Inputs=|+-
  Sum3 : Sum  Inputs=|+-
  Sum4 : Sum  Inputs=++|
  Sum5 : Sum  Inputs=++|
  Sum6 : Sum  Inputs=++|
  Terminator : Terminator
  Terminator1 : Terminator
  Pitch Angle : Outport
  Thrust Control : Outport  Port=2
  wires:
  Desired Energy Evaluator/2(Total Energy Rate Desired) -> Sum5/1, Sum/2
  Gain2/1 -> Sum5/2, Sum1/3
  angle of attack/1 -> Sum4/1
  Actual Energy Evaluator/3(Deficit Energy) -> Sum2/2
  V/1 -> Desired Energy Evaluator/2(V)
  Desired Energy Evaluator/3(Deficit Energy Desired) -> Sum2/1
  Sum3/1 -> Gain2/1
  V_measured/1 -> Gain3/1, Gain/1, Actual Energy Evaluator/2(V)
  Actual Energy Evaluator/4(Total Energy) -> Sum3/2
  h_dot_measured/1 -> Actual Energy Evaluator/3(h_dot)
  Sum/1 -> Sum1/1
  Gain/1 -> Divide/2
  Desired Energy Evaluator/1(Deficit Energy Rate Desired) -> Sum/1
  Gain3/1 -> Divide1/2
  Actual Energy Evaluator/1(Deficit Energy Rate) -> Terminator/1
  Divide1/1 -> Sum6/2
  Actual Energy Evaluator/2(Total Energy Rate) -> Terminator1/1
  h/1 -> Desired Energy Evaluator/4(h)
  Desired Energy Evaluator/4(Total Energy Desired) -> Sum3/1
  Sum5/1 -> Divide1/1
  Sum2/1 -> Gain1/1
  Saturation/1 -> Asin/1
  Gain1/1 -> Sum1/2
  Sum1/1 -> Divide/1
  V_dot_measured/1 -> Actual Energy Evaluator/1(V_dot)
  h_dot/1 -> Desired Energy Evaluator/3(h_dot)
  estimated drag force/1 -> Sum6/1
  V_dot/1 -> Desired Energy Evaluator/1(V_dot)
  Sum6/1 -> Thrust Control/1  "Thrust Control"
  h_measured/1 -> Actual Energy Evaluator/4(h)
  Sum4/1 -> Pitch Angle/1  "Pitch Angle"
  Divide/1 -> Saturation/1
  Asin/1 -> Sum4/2

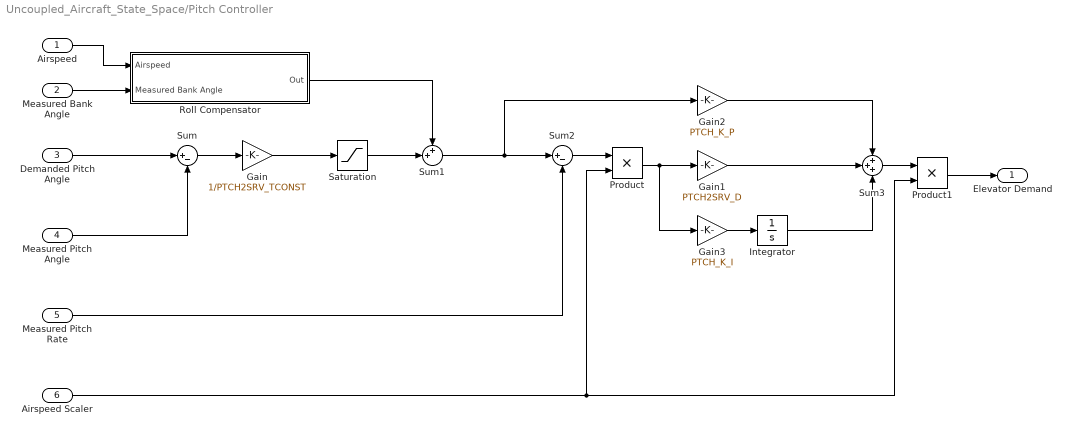
== system Uncoupled_Aircraft_State_Space/Pitch Controller ==
  Airspeed : Inport
  Measured Bank Angle : Inport  Port=2
  Demanded Pitch Angle : Inport  Port=3
  Measured Pitch Angle : Inport  Port=4
  Measured Pitch Rate : Inport  Port=5
  Airspeed Scaler : Inport  Port=6
  Gain : Gain  Gain=1/PTCH2SRV_TCONST
  Gain1 : Gain  Gain=PTCH2SRV_D
  Gain2 : Gain  Gain=PTCH_K_P
  Gain3 : Gain  Gain=PTCH_K_I
  Integrator : Integrator
  Product : Product
  Product1 : Product
  Roll Compensator : Subsystem
  Saturation : Saturate  UpperLimit=PTCH2SRV_RMAX_UP  LowerLimit=PTCH2SRV_RMAX_DN
  Sum : Sum  Inputs=|+-
  Sum1 : Sum  Inputs=++|
  Sum2 : Sum  Inputs=|+-
  Sum3 : Sum  Inputs=+++
  Elevator Demand : Outport
  wires:
  Airspeed/1 -> Roll Compensator/1(Airspeed)
  Gain3/1 -> Integrator/1
  Gain1/1 -> Sum3/2
  Product1/1 -> Elevator Demand/1
  Measured Bank Angle/1 -> Roll Compensator/2(Measured Bank Angle)
  Sum3/1 -> Product1/1
  Measured Pitch Angle/1 -> Sum/2
  Saturation/1 -> Sum1/2
  Sum1/1 -> Gain2/1, Sum2/1
  Product/1 -> Gain3/1, Gain1/1
  Integrator/1 -> Sum3/3
  Demanded Pitch Angle/1 -> Sum/1
  Airspeed Scaler/1 -> Product1/2, Product/2
  Gain/1 -> Saturation/1
  Sum/1 -> Gain/1
  Sum2/1 -> Product/1
  Gain2/1 -> Sum3/1
  Roll Compensator/1(Out) -> Sum1/1
  Measured Pitch Rate/1 -> Sum2/2

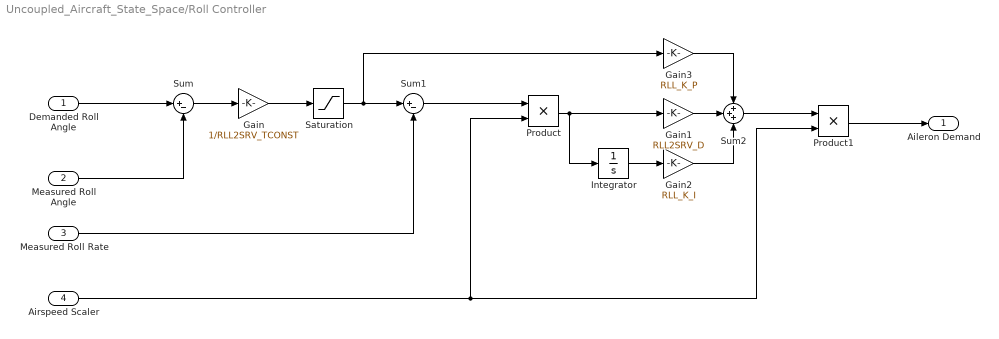
== system Uncoupled_Aircraft_State_Space/Roll Controller ==
  Demanded Roll Angle : Inport
  Measured Roll Angle : Inport  Port=2
  Measured Roll Rate : Inport  Port=3
  Airspeed Scaler : Inport  Port=4
  Gain : Gain  Gain=1/RLL2SRV_TCONST
  Gain1 : Gain  Gain=RLL2SRV_D
  Gain2 : Gain  Gain=RLL_K_I
  Gain3 : Gain  Gain=RLL_K_P
  Integrator : Integrator
  Product : Product
  Product1 : Product
  Saturation : Saturate  UpperLimit=RLL2SRV_MAX  LowerLimit=-RLL2SRV_MAX
  Sum : Sum  Inputs=|+-
  Sum1 : Sum  Inputs=|+-
  Sum2 : Sum  Inputs=+++
  Aileron Demand : Outport
  wires:
  Product/1 -> Integrator/1, Gain1/1
  Sum/1 -> Gain/1
  Saturation/1 -> Sum1/1, Gain3/1
  Gain1/1 -> Sum2/2
  Integrator/1 -> Gain2/1
  Sum2/1 -> Product1/1
  Sum1/1 -> Product/1
  Gain/1 -> Saturation/1
  Gain3/1 -> Sum2/1
  Airspeed Scaler/1 -> Product1/2, Product/2
  Gain2/1 -> Sum2/3
  Demanded Roll Angle/1 -> Sum/1
  Measured Roll Angle/1 -> Sum/2
  Product1/1 -> Aileron Demand/1
  Measured Roll Rate/1 -> Sum1/2

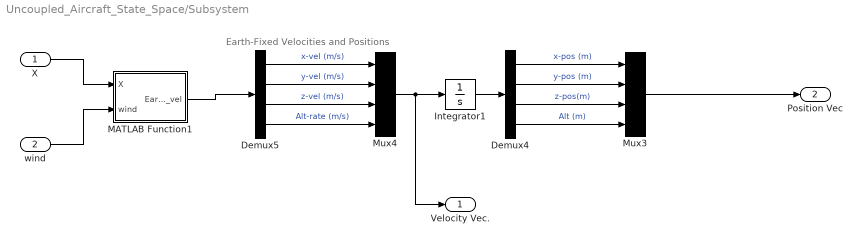
== system Uncoupled_Aircraft_State_Space/Subsystem ==
  note: Earth-Fixed Velocities and Positions
  X : Inport
  wind : Inport  Port=2
  Demux4 : Demux
  Demux5 : Demux
  Integrator1 : Integrator  InitialCondition=[0;0;0;0]
  MATLAB Function1 : MATLAB Function  TreatAsAtomicUnit=on
  Mux3 : Mux
  Mux4 : Mux
  Velocity Vec. : Outport
  Position Vec : Outport  Port=2
  wires:
  Demux4/3 -> Mux3/3  "z-pos(m)"
  Demux4/1 -> Mux3/1  "x-pos (m)"
  Integrator1/1 -> Demux4/1
  Demux4/4 -> Mux3/4  "Alt (m)"
  Mux4/1 -> Velocity Vec./1, Integrator1/1
  Demux5/2 -> Mux4/2  "y-vel (m/s)"
  Demux5/4 -> Mux4/4  "Alt-rate (m/s)"
  Demux5/3 -> Mux4/3  "z-vel (m/s)"
  Demux4/2 -> Mux3/2  "y-pos (m)"
  Mux3/1 -> Position Vec/1
  Demux5/1 -> Mux4/1  "x-vel (m/s)"
  MATLAB Function1/1(Earth_vel) -> Demux5/1
  X/1 -> MATLAB Function1/1(X)
  wind/1 -> MATLAB Function1/2(wind)

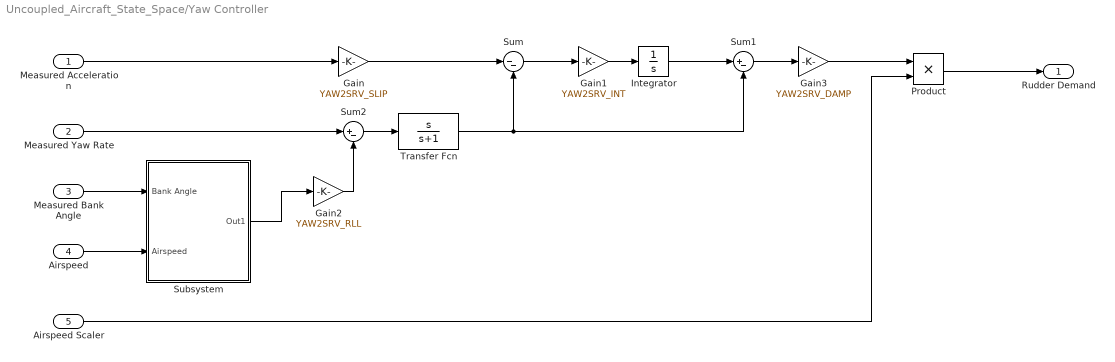
== system Uncoupled_Aircraft_State_Space/Yaw Controller ==
  Measured Acceleration : Inport
  Measured Yaw Rate : Inport  Port=2
  Measured Bank Angle : Inport  Port=3
  Airspeed : Inport  Port=4
  Airspeed Scaler : Inport  Port=5
  Gain : Gain  Gain=YAW2SRV_SLIP
  Gain1 : Gain  Gain=YAW2SRV_INT
  Gain2 : Gain  Gain=YAW2SRV_RLL
  Gain3 : Gain  Gain=YAW2SRV_DAMP
  Integrator : Integrator
  Product : Product
  Subsystem : Subsystem
  Sum : Sum  Inputs=|--
  Sum1 : Sum  Inputs=|+-
  Sum2 : Sum  Inputs=|+-
  Transfer Fcn : TransferFcn  Numerator=[1 0]  Denominator=[1 1]
  Rudder Demand : Outport
  wires:
  Sum1/1 -> Gain3/1
  Gain/1 -> Sum/1
  Gain3/1 -> Product/1
  Subsystem/1(Out1) -> Gain2/1
  Transfer Fcn/1 -> Sum1/2, Sum/2
  Sum/1 -> Gain1/1
  Integrator/1 -> Sum1/1
  Gain2/1 -> Sum2/2
  Measured Acceleration/1 -> Gain/1
  Sum2/1 -> Transfer Fcn/1
  Airspeed/1 -> Subsystem/2(Airspeed)
  Gain1/1 -> Integrator/1
  Measured Bank Angle/1 -> Subsystem/1(Bank Angle)
  Measured Yaw Rate/1 -> Sum2/1
  Airspeed Scaler/1 -> Product/2
  Product/1 -> Rudder Demand/1

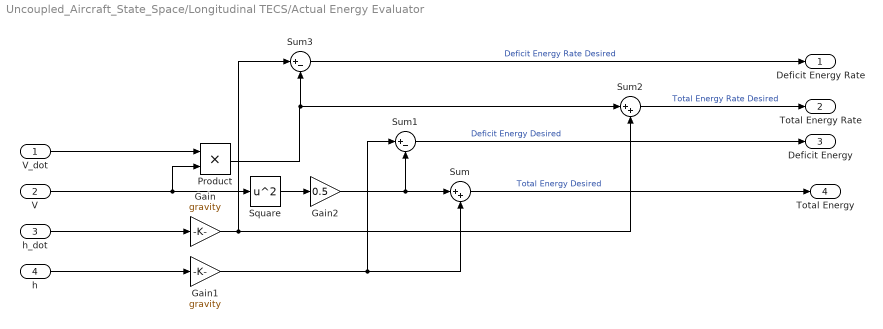
== system Uncoupled_Aircraft_State_Space/Longitudinal TECS/Actual Energy Evaluator ==
  V_dot : Inport
  V : Inport  Port=2
  h_dot : Inport  Port=3
  h : Inport  Port=4
  Gain : Gain  Gain=gravity
  Gain1 : Gain  Gain=gravity
  Gain2 : Gain  Gain=0.5
  Product : Product
  Square : Math  Operator=square
  Sum : Sum  Inputs=|++
  Sum1 : Sum  Inputs=|+-
  Sum2 : Sum  Inputs=|++
  Sum3 : Sum  Inputs=|+-
  Deficit Energy Rate : Outport
  Total Energy Rate : Outport  Port=2
  Deficit Energy : Outport  Port=3
  Total Energy : Outport  Port=4
  wires:
  Gain2/1 -> Sum1/2, Sum/1
  Gain/1 -> Sum3/1, Sum2/2
  Square/1 -> Gain2/1
  Gain1/1 -> Sum1/1, Sum/2
  Product/1 -> Sum2/1, Sum3/2
  V/1 -> Product/2, Square/1
  Sum1/1 -> Deficit Energy/1  "Deficit Energy Desired"
  V_dot/1 -> Product/1
  h_dot/1 -> Gain/1
  h/1 -> Gain1/1
  Sum2/1 -> Total Energy Rate/1  "Total Energy Rate Desired"
  Sum/1 -> Total Energy/1  "Total Energy Desired"
  Sum3/1 -> Deficit Energy Rate/1  "Deficit Energy Rate Desired"

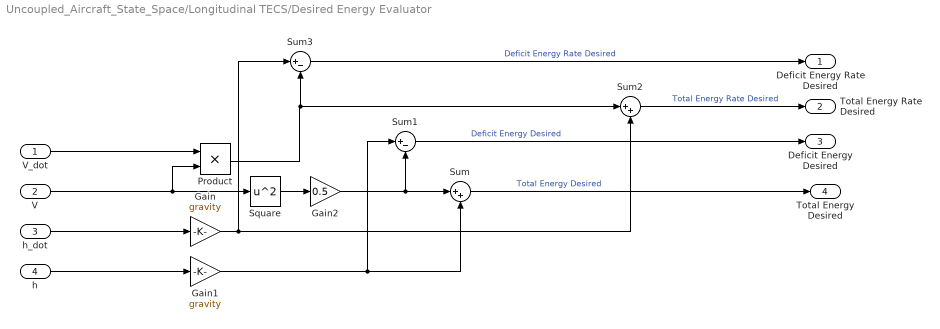
== system Uncoupled_Aircraft_State_Space/Longitudinal TECS/Desired Energy Evaluator ==
  V_dot : Inport
  V : Inport  Port=2
  h_dot : Inport  Port=3
  h : Inport  Port=4
  Gain : Gain  Gain=gravity
  Gain1 : Gain  Gain=gravity
  Gain2 : Gain  Gain=0.5
  Product : Product
  Square : Math  Operator=square
  Sum : Sum  Inputs=|++
  Sum1 : Sum  Inputs=|+-
  Sum2 : Sum  Inputs=|++
  Sum3 : Sum  Inputs=|+-
  Deficit Energy Rate Desired : Outport
  Total Energy Rate Desired : Outport  Port=2
  Deficit Energy Desired : Outport  Port=3
  Total Energy Desired : Outport  Port=4
  wires:
  Gain2/1 -> Sum1/2, Sum/1
  Gain/1 -> Sum3/1, Sum2/2
  Square/1 -> Gain2/1
  Gain1/1 -> Sum1/1, Sum/2
  Product/1 -> Sum2/1, Sum3/2
  V/1 -> Product/2, Square/1
  Sum1/1 -> Deficit Energy Desired/1  "Deficit Energy Desired"
  V_dot/1 -> Product/1
  h_dot/1 -> Gain/1
  h/1 -> Gain1/1
  Sum2/1 -> Total Energy Rate Desired/1  "Total Energy Rate Desired"
  Sum/1 -> Total Energy Desired/1  "Total Energy Desired"
  Sum3/1 -> Deficit Energy Rate Desired/1  "Deficit Energy Rate Desired"

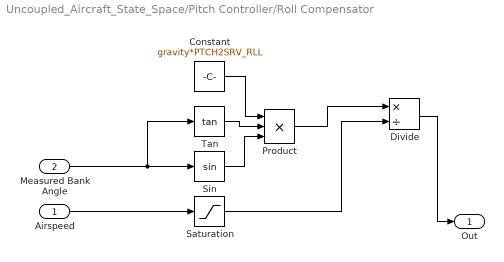
== system Uncoupled_Aircraft_State_Space/Pitch Controller/Roll Compensator ==
  Airspeed : Inport
  Measured Bank Angle : Inport  Port=2
  Constant : Constant  Value=gravity*PTCH2SRV_RLL
  Divide : Product  Inputs=*/
  Product : Product  Inputs=3
  Saturation : Saturate  UpperLimit=inf  LowerLimit=aspd_min
  Sin : Trigonometry
  Tan : Trigonometry  Operator=tan
  Out : Outport
  wires:
  Measured Bank Angle/1 -> Tan/1, Sin/1
  Divide/1 -> Out/1
  Product/1 -> Divide/1
  Tan/1 -> Product/2
  Sin/1 -> Product/3
  Constant/1 -> Product/1
  Airspeed/1 -> Saturation/1
  Saturation/1 -> Divide/2

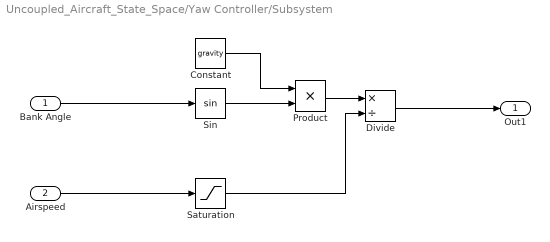
== system Uncoupled_Aircraft_State_Space/Yaw Controller/Subsystem ==
  Bank Angle : Inport
  Airspeed : Inport  Port=2
  Constant : Constant  Value=gravity
  Divide : Product  Inputs=*/
  Product : Product
  Saturation : Saturate  UpperLimit=inf  LowerLimit=aspd_min
  Sin : Trigonometry
  Out1 : Outport
  wires:
  Divide/1 -> Out1/1
  Bank Angle/1 -> Sin/1
  Sin/1 -> Product/2
  Constant/1 -> Product/1
  Product/1 -> Divide/1
  Airspeed/1 -> Saturation/1
  Saturation/1 -> Divide/2

== matlab function Uncoupled_Aircraft_State_Space/MATLAB Function ==
  data: sun_vector input; Euler input; relative_elv output; relative_azimuth output; vec output
function [relative_elv, relative_azimuth,vec] = relative_sun(sun_vector,Euler)


% Sun vector points INTO the aircraft
% It points down when the sun is high
% North at noon in the north hemisphere
% West at sunrise

% Taking the negative (pointing out)

sun_vector = -sun_vector;

% Reformatting into global NED

sun_vector(3) = -sun_vector(3);


% Reframing the sun vector into the body fixed system


pitch = Euler(1);
roll = Euler(2);
heading = Euler(3);


R1E = [ cos(heading),     sin(heading),  0; ...   
        -sin(heading),    cos(heading),  0; ...
        0,                0,             1];

R21 = [ cos(pitch),     0,     -sin(pitch); ...
        0,              1,      0;          ...
        sin(pitch),     0,      cos(pitch)];

RB2 = [ 1,               0,               0; ...
        0,       cos(roll),       sin(roll); ...
        0,      -sin(roll),       cos(roll)];


sun_body_fixed = (RB2*R21*R1E)*sun_vector;
vec = sun_body_fixed;

sx = sun_body_fixed(1);
sy = sun_body_fixed(2);
sz = sun_body_fixed(3);

relative_azimuth = atan2(sy, sx);         % azimuth in xy-plane
relative_elv     = atan2(-sz, hypot(sx,sy)); % use -sz because body z is down




end

== matlab function Uncoupled_Aircraft_State_Space/Subsystem/MATLAB Function1 ==
  data: X input; Earth_vel output; wind input
function Earth_vel = fcn(X,wind)
Earth_vel = zeros(4,1);
Earth_vel1 = zeros(3,1);

Body_vel = [X(1);X(5);X(2)];

roll = X(8);
pitch = X(4);
yaw = X(9);

R_2B = [ 1, 0, 0;
         0, cos(roll), -sin(roll);
         0, sin(roll), cos(roll)];
R_12 = [ cos(pitch), 0, sin(pitch);
         0, 1, 0;
         -sin(pitch),0,cos(pitch)]; 
R_E1 = [ cos(yaw), -sin(yaw), 0;
         sin(yaw), cos(yaw), 0;
         0, 0, 1];

Earth_vel1 = R_E1*R_12*R_2B*Body_vel;

Earth_vel = [Earth_vel1;-Earth_vel1(3)] + [wind;-wind(3)];

== matlab function Uncoupled_Aircraft_State_Space/MATLAB Function1 ==
  data: wpts input; wp_id input; a_cmd output; X input; Y input; Vx input; Vy input; wp_rad input; h_cmd output; ang output; eta_1 output; eta_2 output; CTE output; L1 input; ticker output; rst output
function [a_cmd, h_cmd, ang,eta_1,eta_2,CTE,ticker,rst] = fcn(wpts, wp_id, X, Y, Vx, Vy, wp_rad, L1)

ticker = 0;
rst = 0;
P = [X; Y];                       % Position
V = sqrt(Vx^2 + Vy^2);            % Speed
V_vec = [Vx; Vy];                 % Velocity vector

% --- Waypoint switching ---
A = wpts(1:2, wp_id);   
if (norm(P - A) < wp_rad) && (wp_id < size(wpts, 2) )
    wp_id = wp_id + 1;
    ticker = 1;
end

A_f = wpts(1:2, wp_id);
if (norm(P - A_f) < wp_rad) && (wp_id == size(wpts, 2) )
    rst = 1;
    wp_id = 1;
    ticker = 0;
end

% --- Waypoint anchor and track vector ---
A = wpts(1:2, wp_id);             % Track anchor point
TNG = wpts(4:5, wp_id);           % Track tangent vector

% --- Cross-track error (signed) ---
cross_val = -( (P(1)-A(1))*TNG(2) - (P(2)-A(2))*TNG(1) );
CTE = cross_val / norm(TNG);

% --- Geometric angles ---
eta_1 = asin(max(-1, min(1, CTE / L1)));


cross_TV = TNG(1)*Vy - TNG(2)*Vx;          % 2D “cross”: TNG x V_vec (z-component)
dot_TV   = dot(TNG, V_vec);                % dot product
eta_2 = atan2(cross_TV, dot_TV);           % signed angle in [-pi, pi]

% --- Signed L1 angle ---
ang = eta_2 + sign(cross_val) * abs(eta_1);

% --- Lateral acceleration command ---
a_cmd = 2 * V^2 * sin(ang) / L1;

% --- Altitude command from waypoint table ---
h_cmd = wpts(3, wp_id);

end

== matlab function Uncoupled_Aircraft_State_Space/MATLAB Function2 ==
  data: time_info input; SI output; lat input; long input; alt input
function SI  = solar_vector2(time_info,lat,long,alt)

    % Convert to radians
    lat = deg2rad(lat);
    long = deg2rad(long);

    % Extract time
    YYYY = time_info(1);
    MM   = time_info(2);
    DD   = time_info(3);
    HH   = time_info(4);
    Min  = time_info(5);
    Sec  = time_info(6);

    %% --- Compute "time of year" fraction since winter solstice ---
    % Days from Jan 1 to current date
    current_days = month2days(MM,YYYY) + DD - 1 ...
                   + (HH + (Min + Sec/60)/60) / 24;
    % Days from Jan 1 to winter solstice in previous year (Dec 21)
    solstice_prev = month2days(12,YYYY-1) + 21 - 1;

    % Total days in previous year
    days_prev_year = 365 + leapcomp(YYYY-1);

    % Days since last solstice
    days_since_solstice = current_days + (days_prev_year - solstice_prev);

    % Total days in current year
    days_this_year = 365 + leapcomp(YYYY);

    % Fraction of year since solstice
    ToY = days_since_solstice / days_this_year;

    % Orbital angle
    angle_in_orbit = -(2*pi)*(ToY);

    %% --- Geometry ---
    % Earth radius with altitude
    R_e = 6.371e6 + alt;

    % Solar vector in orbital frame
    S_vec = [cos(angle_in_orbit), sin(angle_in_orbit), 0];
    S_vec = S_vec / norm(S_vec);

    % Position on Earth surface
    P = R_e * [cos(lat)*cos(long), cos(lat)*sin(long), sin(lat)];

    % Earth axis tilt
    tilt = deg2rad(-23.5);
    a = [sin(tilt), 0, cos(tilt)];
    north_pole = a';

    q1 = quaternion([cos(tilt/2), 0, sin(tilt/2), 0]);

    %% --- Time of day rotation ---
    % Fraction of current day
    frac_day = (HH + Min/60 + Sec/3600) / 24;

    % This matches: theta = 2*pi*days(time_info-ref_D)
    theta = 2*pi*frac_day + angle_in_orbit + pi;

    % Rotations
    q2 = quaternion([cos(theta/2), sin(theta/2)*a]);
    q_total = q2 * q1;

    % Position in ECEF
    r = rotatepoint(q_total, P)';

    % Up vector
    up = r / norm(r);

    % North vector
    north = north_pole - (dot(north_pole, up) * up);
    north = north / norm(north);

    % East vector
    east = cross(north, up);

    % Solar vector components in NEU
    SI = [dot(S_vec, north) / norm(north);
          dot(S_vec, east)  / norm(east);
          dot(S_vec, up)    / norm(up)];

    SI = -SI;
end


%% Helper: cumulative days until given month
function days = month2days(months,year)
    days_in_month = [31,28,31,30,31,30,31,31,30,31,30,31];
    if leapcomp(year)
        days_in_month(2) = 29;
    end
    days = sum(days_in_month(1:months-1));
end

%% Helper: leap year check
function comp = leapcomp(year)
    comp = (mod(year,4) == 0 && (mod(year,100) ~= 0 || mod(year,400) == 0));
end

== matlab function Uncoupled_Aircraft_State_Space/MATLAB Function3 ==
  data: Earth_Wind input; Wind output; X input
function Wind = fcn(Earth_Wind,X)


Wind = zeros(3,1);

roll = X(8);
pitch = X(4);
yaw = X(9);

R_B2 = [ 1, 0, 0;
         0, cos(roll), sin(roll);
         0, -sin(roll), cos(roll)];

R_21 = [ cos(pitch), 0, -sin(pitch);
         0,          1,           0;
         sin(pitch), 0,  cos(pitch)]; 

R_1E = [ cos(yaw), sin(yaw), 0;
         -sin(yaw), cos(yaw), 0;
         0, 0, 1];

Wind = (R_B2*R_21*R_1E)*Earth_Wind;

== matlab function Uncoupled_Aircraft_State_Space/MATLAB Function4 ==
  data: lat_deg input; lat_rate_deg output; lon_deg input; h input; neu_vel input; lon_rate_deg output; h_rate output
function [lat_rate_deg, lon_rate_deg, h_rate] = neu_vel_to_rates(lat_deg, lon_deg, h, neu_vel)
% neu_vel_to_rates  Convert NEU velocities into geodetic rates
%
% Inputs:
%   lat_deg   - current latitude (deg)
%   lon_deg   - current longitude (deg)   (not needed here, but useful for completeness)
%   h         - current altitude (m)
%   neu_vel   - [vN; vE; vU] velocities (m/s)
%
% Outputs:
%   lat_rate_deg - latitude rate (deg/s)
%   lon_rate_deg - longitude rate (deg/s)
%   h_rate       - altitude rate (m/s)

% WGS-84 constants
a = 6378137.0;             
f = 1/298.257223563;       
e2 = f*(2-f);

% Convert latitude to radians
lat = deg2rad(lat_deg);

% Radii of curvature
N = a / sqrt(1 - e2*sin(lat)^2);             
M = a*(1 - e2) / (1 - e2*sin(lat)^2)^(3/2);

% Extract NEU velocities
vN = neu_vel(1);
vE = neu_vel(2);
vU = neu_vel(3);

% Convert velocities to angular rates
lat_rate = vN / (M + h);                      % rad/s
lon_rate = vE / ((N + h) * cos(lat));         % rad/s
h_rate   = vU;                                % m/s

% Convert angular rates to deg/s
lat_rate_deg = rad2deg(lat_rate);
lon_rate_deg = rad2deg(lon_rate);

end
